simulink model "two_loop_stering_v24"  (R2019b)
settings: Solver=VariableStepAuto  StartTime=0  StopTime=8000  FixedStep=1  MaxStep=1.5  MinStep=0.5  RelTol=1
undefined symbols (not defined in the file or in its folder): sigbuilder_block
libraries: mpclib x1
settings Model: SimulationMode=accelerator  Creator=kuba9  LastModifiedBy=Jakub
settings SolverCC: InitialStep=1

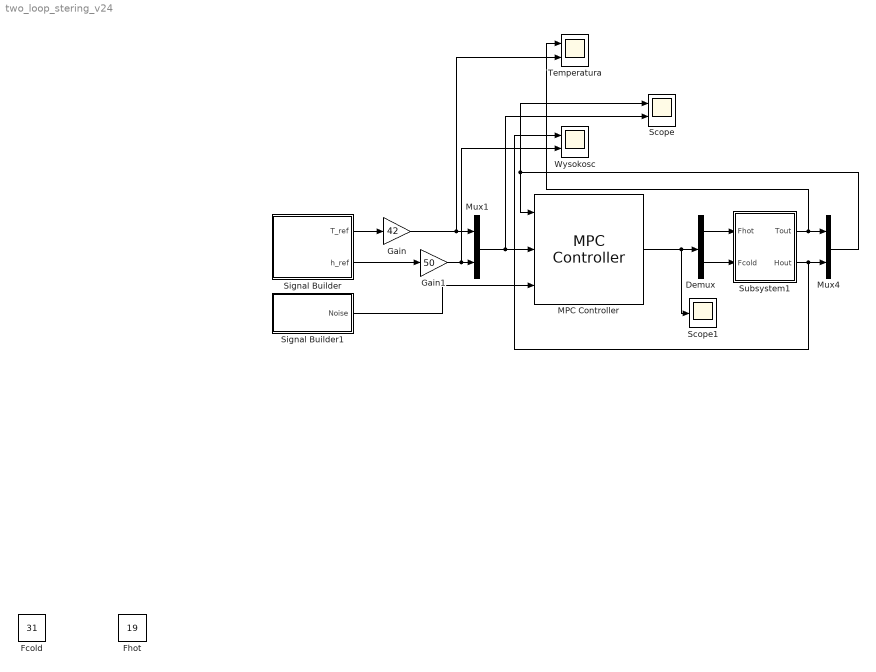
== system two_loop_stering_v24 ==
  Demux : Demux  Outputs=2
  "Fcold " : Constant  Value=31
  "Fhot " : Constant  Value=19
  Gain : Gain  Gain=42
  Gain1 : Gain  Gain=50
  MPC Controller : mpclib/MPC Controller  SCDEnableBlockLinearizationSpecification=on  mpcobj=mpc1  is_multiple=0  enable_value=0  return_u0=off  updateMPCinCallerWorkspace=on  md_inport=on  mv_inport=off  uref_inport=off  return_cost=off  return_mvseq=off  return_qpstatus=off  return_xseq=off  return_state=off  return_ovseq=off  state_inport=off  umin_inport=off  umax_inport=off  ymin_inport=off  ymax_inport=off  cc_inport=off  ywt_inport=off  uwt_inport=off  duwt_inport=off  rhoeps_inport=off  pm_inport=off  MaximumP=10  HorizonChoice=FixedHorizon  n_ts=1  n_p=10  n_mv=2  n_md=1  n_ud=0  n_mo=2  n_uo=0  BlockDataType=double  SampleTimeInherited=off  switch_inport=off
  Mux1 : Mux  Inputs=2
  Mux4 : Mux  Inputs=2
  Scope : Scope  NumInputPorts=2
  Scope1 : Scope
  Signal Builder : Subsystem  Tag=STV Subsys  LoadFcn=sigbuilder_block('load');  StartFcn=sigbuilder_block('start');  StopFcn=sigbuilder_block('stop');  ClipboardFcn=sigbuilder_block('clipboard');  mask(Sigbuilder block){tuvar=[0:10]}
      mask help: Simulink:masks:SigbuilderBlock_MD
      mask init:
      | if ~strcmp(get_param(bdroot(gcbh),'SimulationStatus'),'stopped') tuvar = sigbuilder_block('maskInit'); end
      settings: CopyFcn=sigbuilder_block('copy');  DeleteFcn=sigbuilder_block('delete');  ModelCloseFcn=sigbuilder_block('modelClose');  PreSaveFcn=sigbuilder_block('preSave');  PauseFcn=sigbuilder_block('pause');  ContinueFcn=sigbuilder_block('continue');  NameChangeFcn=sigbuilder_block('namechange');  OpenFcn=sigbuilder_block('open',[81 206.25 1012.5 447.75 ]);  CloseFcn=sigbuilder_block('close');
      mask Display: plot(0, 0, 100, 100,[2, 2, 32, 32, 2], [68, 8, 8, 68, 68],[32, 2], [38, 38], [32, 19, 2],[53, 60, 44], [32, 17, 17, 2],[16, 16, 31, 31]);txt = getActiveGroup(gcbh);text(2, 100, txt,'verticalAlignment', 'top');
  Signal Builder1 : Subsystem  Tag=STV Subsys  LoadFcn=sigbuilder_block('load');  StartFcn=sigbuilder_block('start');  StopFcn=sigbuilder_block('stop');  ClipboardFcn=sigbuilder_block('clipboard');  mask(Sigbuilder block){tuvar=[0:10]}
      mask help: Simulink:masks:SigbuilderBlock_MD
      mask init:
      | if ~strcmp(get_param(bdroot(gcbh),'SimulationStatus'),'stopped') tuvar = sigbuilder_block('maskInit'); end
      settings: CopyFcn=sigbuilder_block('copy');  DeleteFcn=sigbuilder_block('delete');  ModelCloseFcn=sigbuilder_block('modelClose');  PreSaveFcn=sigbuilder_block('preSave');  PauseFcn=sigbuilder_block('pause');  ContinueFcn=sigbuilder_block('continue');  NameChangeFcn=sigbuilder_block('namechange');  OpenFcn=sigbuilder_block('open',[172.5 199.2 1143 400 ]);  CloseFcn=sigbuilder_block('close');
      mask Display: plot(0, 0, 100, 100,[2, 2, 32, 32, 2], [68, 8, 8, 68, 68],[32, 2], [38, 38], [32, 19, 2],[53, 60, 44], [32, 17, 17, 2],[16, 16, 31, 31]);txt = getActiveGroup(gcbh);text(2, 100, txt,'verticalAlignment', 'top');
  Subsystem1 : Subsystem
  Temperatura : Scope  NumInputPorts=2
  Wysokosc : Scope  NumInputPorts=2
  wires:
  Signal Builder/2(h_ref) -> Gain1/1
  Signal Builder/1(T_ref) -> Gain/1
  Gain1/1 -> Wysokosc/2, Mux1/2
  Subsystem1/1(Tout) -> Mux4/1, Temperatura/1
  Subsystem1/2(Hout) -> Wysokosc/1, Mux4/2
  MPC Controller/1 -> Scope1/1, Demux/1
  Mux4/1 -> MPC Controller/1, Scope/1
  Gain/1 -> Temperatura/2, Mux1/1
  Mux1/1 -> MPC Controller/2, Scope/2
  Demux/1 -> Subsystem1/1("Fhot ")
  Demux/2 -> Subsystem1/2("Fcold ")
  Signal Builder1/1(Noise) -> MPC Controller/3

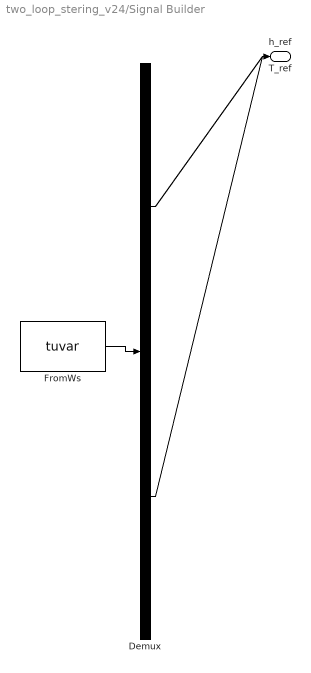
== system two_loop_stering_v24/Signal Builder ==
  Demux : Demux  Tag=STV Demux  Outputs=2
  FromWs : FromWorkspace  Tag=STV FromWs  VariableName=tuvar  SampleTime=0
      SigBuilderData=|
      | common.afterFinalStr = 'Extrapolate'
      | common.sampleTime = 0
      | dataSet.timeRange = [0 8000]
      | dataSet.name = 'Group 1'
      | sbobj.Groups.Name = 'Group 1'
      | sbobj.Groups.Signals(1).Name = 'T_ref'
      | sbobj.Groups.Signals(1).XData = [0 2000 3000 4460 5000 6000 8000]
      | sbobj.Groups.Signals(1).YData = [1 1 0.8 0.8 0.8 0.7 0.7]
      | sbobj.Groups.Signals(2).Name = 'h_ref'
      | sbobj.Groups.Signals(2).XData = [0 1000 1100 3100 3600 8000]
      | sbobj.Groups.Signals(2).YData = [1 1 1.2 1.2 1 1]
      | sbobj.Groups.TimeRange = [0 8000]
  T_ref : Outport  Tag=STV Outport
  h_ref : Outport  Tag=STV Outport  Port=2
  wires:
  FromWs/1 -> Demux/1
  Demux/1 -> T_ref/1
  Demux/2 -> h_ref/1

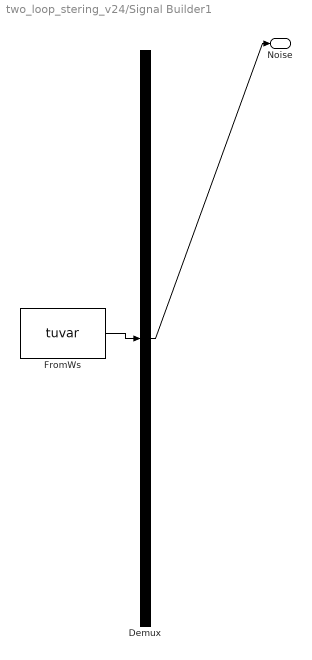
== system two_loop_stering_v24/Signal Builder1 ==
  Demux : Demux  Tag=STV Demux  Outputs=1
  FromWs : FromWorkspace  Tag=STV FromWs  VariableName=tuvar  SampleTime=0
      SigBuilderData=|
      | common.afterFinalStr = 'Extrapolate'
      | common.sampleTime = 0
      | dataSet.timeRange = [0 8000]
      | dataSet.name = 'Group 1'
      | sbobj.Groups.Name = 'Group 1'
      | sbobj.Groups.Signals.Name = 'Noise'
      | sbobj.Groups.Signals.XData = [0 10 10 30 30 50 50 60 60 80 80 90 ... (802 elements, 1x802)]
      | sbobj.Groups.Signals.YData = [0.05 0.05 0.7 0.7 0.05 0.05 0.7 0.7 0.05 0.05 0.7 0.7 ... (802 elements, 1x802)]
      | sbobj.Groups.TimeRange = [0 8000]
  Noise : Outport  Tag=STV Outport
  wires:
  FromWs/1 -> Demux/1
  Demux/1 -> Noise/1

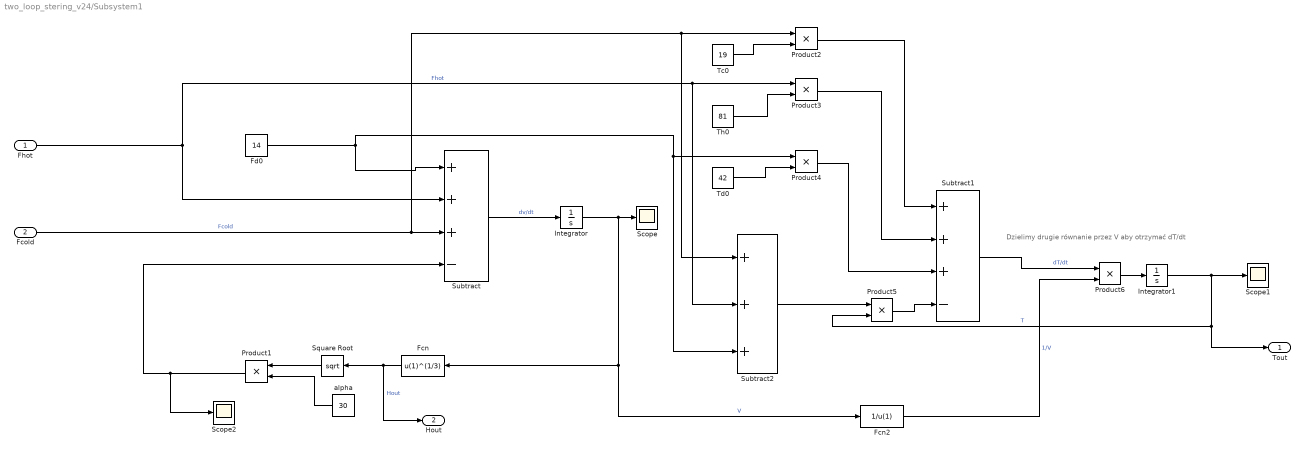
== system two_loop_stering_v24/Subsystem1 ==
  note: Dzielimy drugie równanie przez V aby otrzymać dT/dt
  "Fhot " : Inport
  "Fcold " : Inport  Port=2
  Fcn : Fcn  Expr=u(1)^(1/3)
  Fcn2 : Fcn  Expr=1/u(1)
  Fd0 : Constant  Value=14
  Integrator : Integrator  InitialCondition=125000  ZeroCross=off
  Integrator1 : Integrator  InitialCondition=42
  Product{1..6} (6 alike) : Product
  Scope : Scope
  Scope1 : Scope
  Scope2 : Scope
  Square Root : Sqrt  SaturateOnIntegerOverflow=on
  Subtract : Sum  Inputs=+++-
  Subtract1 : Sum  Inputs=+++-
  Subtract2 : Sum  Inputs=+++
  Tc0 : Constant  Value=19
  Td0 : Constant  Value=42
  Th0 : Constant  Value=81
  alpha : Constant  Value=30
  Tout : Outport
  Hout : Outport  Port=2
  wires:
  "Fcold "/1 -> Subtract2/1, Product2/1, Subtract/3  "Fcold"
  Integrator/1 -> Fcn/1, Fcn2/1, Scope/1  "V"
  alpha/1 -> Product1/2
  Fd0/1 -> Subtract/1, Subtract2/3, Product4/1
  Th0/1 -> Product3/2
  Td0/1 -> Product4/2
  Product2/1 -> Subtract1/1
  Fcn/1 -> Hout/1, Square Root/1  "Hout"
  "Fhot "/1 -> Subtract/2, Subtract2/2, Product3/1  "Fhot"
  Tc0/1 -> Product2/2
  Integrator1/1 -> Product5/2, Tout/1, Scope1/1  "T"
  Subtract/1 -> Integrator/1  "dv/dt"
  Subtract1/1 -> Product6/1  "dT/dt"
  Product4/1 -> Subtract1/3
  Subtract2/1 -> Product5/1
  Product6/1 -> Integrator1/1
  Product3/1 -> Subtract1/2
  Product5/1 -> Subtract1/4
  Fcn2/1 -> Product6/2  "1/V"
  Square Root/1 -> Product1/1
  Product1/1 -> Scope2/1, Subtract/4
